simulink model "collision_avoidance_260310"  (R2024b)
settings: Solver=FixedStepAuto  StartTime=0.0  StopTime=inf  RelTol=1e-3  EnableMultiTasking=on
values from neighbouring files (symbols this model uses):
  Fx_max = 1    [Init_collision_avoidance_UGV.m]
  Fx_min = -1    [Init_collision_avoidance_UGV.m]
  N_max = 1    [Init_collision_avoidance_UGV.m]
  N_min = -1    [Init_collision_avoidance_UGV.m]
  RC_max = 2000    [Init_collision_avoidance_UGV.m]
  RC_min = 1000    [Init_collision_avoidance_UGV.m]
  ref_lla = [36.365227, 127.345838, 25.1110]    [Init_collision_avoidance_UGV.m]
undefined symbols (not defined in the file or in its folder): DiscIntNeverNeededParam, modeeight, modefive, modefour, modenine, modeone, modeseven, modesix, modeten, modethree, modetwo, motor_pwm_time_log, psi_time_log, r_time_log, rc_on_off, steering_pwm_time_log, taun_time_log, taux_time_log, timestamp, u_time_log, v_time_log, x_time_log, y_time_log
libraries: px4uORBlib x14, px4Utilslib x9, sharedtransform x2, sharedutil x1, px4Peripheralslib x1, px4Sensorslib x1
settings Model: ExtModeTrigDuration=10  Creator=ADMIN  LastModifiedBy=User
settings SolverCC: PositivePriorityOrder=on
settings OptimizationCC: EnhancedBackFolding=on  PassReuseOutputArgsAs=Individual arguments  ZeroExternalMemoryAtStartup=off  ZeroInternalMemoryAtStartup=off  MaxStackSize=64  OptimizeBlockOrder=speed  DifferentSizesBufferReuse=on  OptimizationCustomize=off  EfficientTunableParamExpr=on
settings DebuggingCC: ParameterTunabilityLossMsg=error
settings HardwareCC: ProdBitPerPointer=32  ProdBitPerSizeT=32  ProdBitPerPtrDiffT=32  ProdLargestAtomicInteger=Long  ProdLargestAtomicFloat=Double  ProdWordSize=32  ProdLongLongMode=on  ProdHWDeviceType=ARM Compatible->ARM Cortex
settings SFSimCC: MATLABDynamicMemAlloc=off  SimTargetLang=C++
settings RTWCC: Description=Embedded Coder  SystemTargetFile=ert.tlc  HardwareBoard=PX4 Pixhawk 6x  TLCOptions="-aInlineSetEventsForThisBaseRateFcn=TLC_FALSE -aSuppressMultiTaskScheduler=TLC_FALSE  -aRateBasedStepFcn=0"  TemplateMakefile=ert_default_tmf  Toolchain=GNU Tools for PX4 Autopilots  TargetLang=C++  GPUComputeCapability=3.5
settings CodeAppCC: ForceParamTrailComments=on  IgnoreCustomStorageClasses=off  OperatorAnnotations=on  SimulinkDataObjDesc=on  SFDataObjDesc=on  InsertBlockDesc=on
settings ERTTargetCC: ExtModeTransport=3  ExtModeStaticAlloc=on  ExtModeStaticAllocSize=1024  ExtModeMexFile=ext_xcp  ExtModeIntrfLevel=Level2 - Open  InlinedParameterPlacement=Hierarchical  DynamicArrayContainerType=coder::array

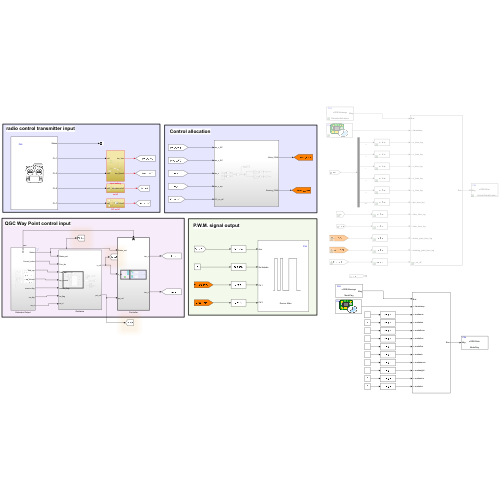
[thumbnail: Simulink's stored preview of the top-level diagram]
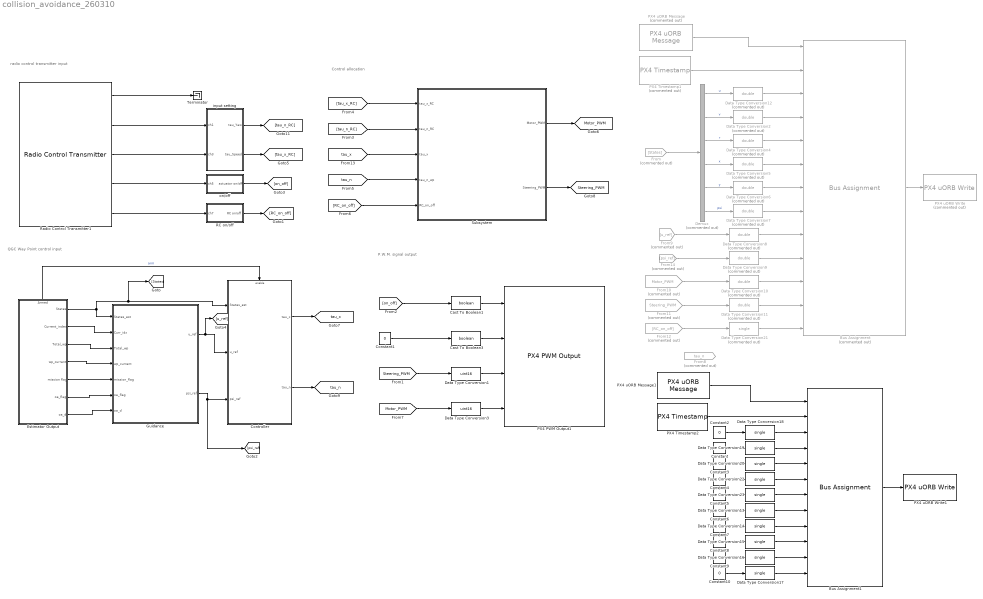
== system collision_avoidance_260310 ==
  note: radio control transmitter input
  note: P.W.M. signal output
  note: Control allocation
  note: QGC Way Point control input
  Bus Assignment : BusAssignment  Commented=on  AssignedSignals=timestamp,u_time_log,v_time_log,r_time_log,x_time_log,y_time_log,psi_time_log,taux_time_log,taun_time_log,motor_pwm_time_log,steering_pwm_time_log,rc_on_off
  Bus Assignment1 : BusAssignment  AssignedSignals=timestamp,modeone,modetwo,modethree,modefour,modefive,modesix,modeseven,modeeight,modenine,modeten
  Cast To Boolean1 : DataTypeConversion  OutDataTypeStr=boolean  SaturateOnIntegerOverflow=off  RndMeth=Floor
  Cast To Boolean3 : DataTypeConversion  OutDataTypeStr=boolean  SaturateOnIntegerOverflow=off  RndMeth=Floor
  Constant : Constant
  Constant{1..10} (10 alike) : Constant  Value=0
  Controller : Subsystem
  Data Type Conversion1 : DataTypeConversion  OutDataTypeStr=uint16  SaturateOnIntegerOverflow=off  RndMeth=Floor
  Data Type Conversion{2,4..12} (10 alike) : DataTypeConversion  Commented=on  OutDataTypeStr=double  RndMeth=Nearest  SaturateOnIntegerOverflow=off
  Data Type Conversion{13..20,22..23} (10 alike) : DataTypeConversion  OutDataTypeStr=single  RndMeth=Nearest  SaturateOnIntegerOverflow=off
  Data Type Conversion21 : DataTypeConversion  Commented=on  OutDataTypeStr=single  RndMeth=Nearest  SaturateOnIntegerOverflow=off
  Data Type Conversion3 : DataTypeConversion  OutDataTypeStr=uint16  SaturateOnIntegerOverflow=off  RndMeth=Floor
  Demux : Demux  Commented=on  Outputs=6
  Estimator Output : Subsystem
      settings: PortSchema="{\"entries\":[{\"content\":{\"sides\":[{\"content\":{},\"type\":\"ConnectorPlacement.EquallySpacedRectSide\",\"uuid\":\"1d36fcc8-80dd-4f77-9fb4-99d02af10106\"},{\"content\":{\"connectorIds\":[\"Out1\",\"Out2\",\"Out3\",\"Out4\",\"Out5\",\"Out6\",\"Out7\"],\"side\":\"RIGHT\"},\"type\":\"ConnectorPlacement.EquallySpacedRectSide\",\"uuid\":\"b131ae5f-f834-4065-827d-4788e597b476\"},{\"content\":{\"connectorIds\":[\"Out8\"],\"side\":\"TOP\"},\"type\":\"ConnectorPlacement.EquallySpacedRectSide\",\"uuid\":\"02aebafc-cadb-49e7-bb89-79250ef56f49\"}]},\"type\":\"ConnectorPlacement.EquallySpacedConnector\",\"uuid\":\"ac2ee399-74d4-4a66-adbe-2c3e3c8a8081\"}],\"packageUris\":[\"http://schema.mathworks.com/mf0/Connector/R2020b\"],\"version\":\"1.0\"}"
  From : From  Commented=on  GotoTag=States
  From10 : From  Commented=on  GotoTag=Motor_PWM  TagVisibility=global
  From11 : From  Commented=on  GotoTag=Steering_PWM  TagVisibility=global
  From12 : From  Commented=on  GotoTag=RC_on_off
  From14 : From  Commented=on  GotoTag=psi_ref
  From8 : From  Commented=on  GotoTag=tau_n  TagVisibility=global
  From9 : From  Commented=on  GotoTag=u_ref
  "Guidance " : Subsystem
  PX4 PWM Output1 : px4Peripheralslib/PX4 PWM Output  pwmDevice=Main  pwmChannel1_=on  pwmChannel2_=off  pwmChannel3_=on  pwmChannel4_=off  pwmChannel5_=off  pwmChannel6_=off  pwmChannel7_=off  pwmChannel8_=off
      settings: SourceProductName=PX4 Peripheral Blocks
  PX4 Timestamp1 : px4Utilslib/PX4 Timestamp  Commented=on  SampleTime=-1
      settings: SourceProductName=PX4 Utility Blocks
  PX4 Timestamp2 : px4Utilslib/PX4 Timestamp  SampleTime=-1
      settings: SourceProductName=PX4 Utility Blocks
  PX4 uORB Message : px4uORBlib/PX4 uORB Message  Commented=on  uORBTopic=StatesAndActuators  SampleTime=-1  selectInstance=StatesAndActuators
  PX4 uORB Message1 : px4uORBlib/PX4 uORB Message  uORBTopic=ModeFlag  SampleTime=-1  selectInstance=ModeFlag
  PX4 uORB Write : px4uORBlib/PX4 uORB Write  Commented=on  uORBTopic=VehicleGlobalPosition  selectInstance=vehicle_global_position  MessageQueueLen=1
  PX4 uORB Write1 : px4uORBlib/PX4 uORB Write  uORBTopic=ModeFlag  selectInstance=ModeFlag  MessageQueueLen=1
  RC on/off : Subsystem
  Radio Control Transmitter1 : px4Sensorslib/Radio Control Transmitter  channel1=on  channel2=off  channel3=on  channel4=off  channel5=on  channel6=off  channel7=on  channel8=off  channel_count=off  rssi=off  rc_input_source=off  timestamp_last_signal=off  time_stamp=off  sampleTime=1/250  BlockingMode=off  BlockTimeout=5
  Subsystem : Subsystem
  Terminator : Terminator
  input setting : Subsystem
  on/off : Subsystem
  tag scope: Motor_PWM=global, Steering_PWM=global, tau_n=global, tau_x=global
  wires:
  [tau_n_RC] -> Subsystem/2(tau_n_RC)
  Radio Control Transmitter1/3 -> input setting/2(ch3)
  on/off/1(actuator on/off) -> [on_off]
  Radio Control Transmitter1/1 -> Terminator/1
  Radio Control Transmitter1/4 -> on/off/1(ch5)
  [on_off] -> Cast To Boolean1/1
  Constant1/1 -> Cast To Boolean3/1
  Radio Control Transmitter1/5 -> RC on/off/1(ch7)
  RC on/off/1(RC on/off) -> [RC_on_off]
  input setting/1(tau_Yaw) -> [tau_n_RC]
  input setting/2(tau_Speed) -> [tau_x_RC]
  Radio Control Transmitter1/2 -> input setting/1(ch1)
  [tau_x] -> Subsystem/3(tau_x)
  [RC_on_off] -> Subsystem/5(RC_on_off)
  [tau_n] -> Subsystem/4(tau_n_wp)
  Cast To Boolean1/1 -> PX4 PWM Output1/1
  Cast To Boolean3/1 -> PX4 PWM Output1/2
  Data Type Conversion1/1 -> PX4 PWM Output1/3
  Data Type Conversion3/1 -> PX4 PWM Output1/4
  Subsystem/1(Motor_PWM) -> [Motor_PWM]
  Subsystem/2(Steering_PWM) -> [Steering_PWM]
  [Steering_PWM] -> Data Type Conversion1/1
  [Motor_PWM] -> Data Type Conversion3/1
  Estimator Output/4(wp_current) -> "Guidance "/4(wp_current)
  Estimator Output/3(Total_wp) -> "Guidance "/3(Total_wp)
  Estimator Output/2(Current_index) -> "Guidance "/2(Curr_idx)
  Estimator Output/1(States) -> [States], Controller/1(States_est), "Guidance "/1(States_est)
  Estimator Output/5(mission flag) -> "Guidance "/5(mission_flag)
  "Guidance "/1(u_ref) -> Controller/2(u_ref), [u_ref]
  "Guidance "/2(psi_ref) -> [psi_ref], Controller/3(psi_ref)
  Controller/2(tau_n) -> [tau_n]
  Controller/1(tau_x) -> [tau_x]
  [tau_x_RC] -> Subsystem/1(tau_x_RC)
  Estimator Output/8(Armed) -> Controller/Enable  "arm"
  From/1 -> Demux/1
  Demux/1 -> Data Type Conversion12/1  "u"
  Demux/2 -> Data Type Conversion2/1  "v"
  Demux/3 -> Data Type Conversion4/1  "r"
  Demux/4 -> Data Type Conversion5/1  "x"
  Demux/5 -> Data Type Conversion6/1  "y"
  Demux/6 -> Data Type Conversion7/1  "psi"
  From9/1 -> Data Type Conversion8/1
  From14/1 -> Data Type Conversion9/1
  From10/1 -> Data Type Conversion10/1
  From11/1 -> Data Type Conversion11/1
  Constant6/1 -> Data Type Conversion13/1
  Data Type Conversion23/1 -> Bus Assignment1/7
  Constant8/1 -> Data Type Conversion15/1
  Constant9/1 -> Data Type Conversion16/1
  Data Type Conversion19/1 -> Bus Assignment1/4
  Data Type Conversion15/1 -> Bus Assignment1/10
  Constant/1 -> Data Type Conversion19/1
  Data Type Conversion16/1 -> Bus Assignment1/11
  Constant2/1 -> Data Type Conversion18/1
  Constant3/1 -> Data Type Conversion20/1
  Data Type Conversion17/1 -> Bus Assignment1/12
  Data Type Conversion18/1 -> Bus Assignment1/3
  Data Type Conversion13/1 -> Bus Assignment1/8
  Data Type Conversion14/1 -> Bus Assignment1/9
  Data Type Conversion22/1 -> Bus Assignment1/6
  Constant5/1 -> Data Type Conversion23/1
  Constant4/1 -> Data Type Conversion22/1
  Constant7/1 -> Data Type Conversion14/1
  Constant10/1 -> Data Type Conversion17/1
  Data Type Conversion20/1 -> Bus Assignment1/5
  PX4 uORB Message/1 -> Bus Assignment/1
  PX4 Timestamp1/1 -> Bus Assignment/2
  From12/1 -> Data Type Conversion21/1
  Data Type Conversion11/1 -> Bus Assignment/12
  Data Type Conversion10/1 -> Bus Assignment/11
  Data Type Conversion9/1 -> Bus Assignment/10
  Data Type Conversion8/1 -> Bus Assignment/9
  Data Type Conversion7/1 -> Bus Assignment/8
  Data Type Conversion6/1 -> Bus Assignment/7
  Data Type Conversion5/1 -> Bus Assignment/6
  Data Type Conversion4/1 -> Bus Assignment/5
  Data Type Conversion2/1 -> Bus Assignment/4
  Data Type Conversion12/1 -> Bus Assignment/3
  Bus Assignment/1 -> PX4 uORB Write/1
  PX4 uORB Message1/1 -> Bus Assignment1/1
  PX4 Timestamp2/1 -> Bus Assignment1/2
  Bus Assignment1/1 -> PX4 uORB Write1/1
  Estimator Output/6(oa_flag) -> "Guidance "/6(oa_flag)
  Estimator Output/7(oa_d) -> "Guidance "/7(oa_d)
  Data Type Conversion21/1 -> Bus Assignment/13

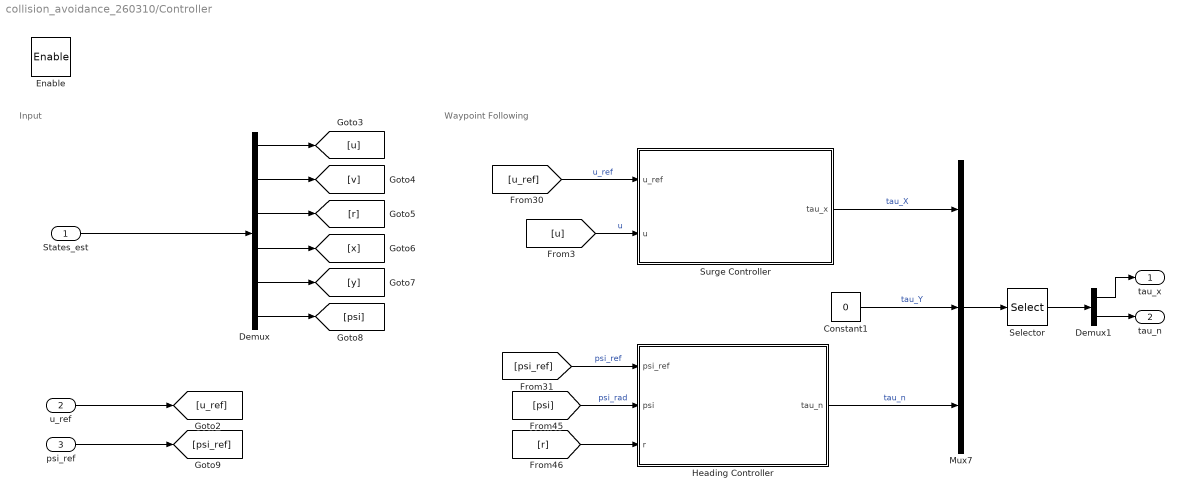
== system collision_avoidance_260310/Controller ==
  note: Input
  note: Waypoint Following
  States_est : Inport
  u_ref : Inport  Port=2
  psi_ref : Inport  Port=3
  Enable : EnablePort
  Constant1 : Constant  Value=0
  Demux : Demux  Outputs=6
  Demux1 : Demux  Outputs=2
  Heading Controller : Subsystem
  Mux7 : Mux  Inputs=3
  Selector : Selector  InputPortWidth=3  IndexOptions=Index vector (dialog)  Indices=[1 3]  OutputSizes=1
  Surge Controller : Subsystem
  tau_x : Outport
  tau_n : Outport  Port=2
  wires:
  Surge Controller/1(tau_x) -> Mux7/1  "tau_X"
  Constant1/1 -> Mux7/2  "tau_Y"
  [psi_ref] -> Heading Controller/1(psi_ref)  "psi_ref"
  [r] -> Heading Controller/3(r)
  Mux7/1 -> Selector/1
  States_est/1 -> Demux/1
  Demux/1 -> [u]
  Demux/2 -> [v]
  Demux/3 -> [r]
  Demux/4 -> [x]
  Demux/5 -> [y]
  Demux/6 -> [psi]
  u_ref/1 -> [u_ref]
  psi_ref/1 -> [psi_ref]
  [u_ref] -> Surge Controller/1(u_ref)  "u_ref"
  [u] -> Surge Controller/2(u)  "u"
  Heading Controller/1(tau_n) -> Mux7/3  "tau_n"
  [psi] -> Heading Controller/2(psi)  "psi_rad"
  Selector/1 -> Demux1/1
  Demux1/1 -> tau_x/1
  Demux1/2 -> tau_n/1

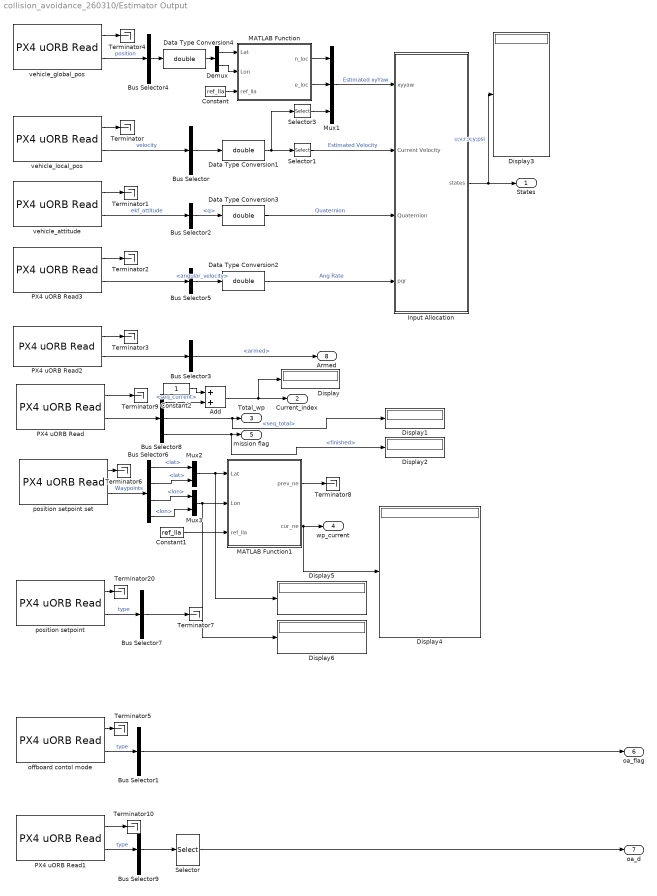
== system collision_avoidance_260310/Estimator Output ==
  Add : Sum
  Bus Selector : BusSelector  OutputSignals=vx,vy,vz,heading  OutputAsBus=on
  Bus Selector1 : BusSelector  OutputSignals=position,velocity,attitude  OutputAsBus=on
  Bus Selector2 : BusSelector  OutputSignals=q
  Bus Selector3 : BusSelector  OutputSignals=armed
  Bus Selector4 : BusSelector  OutputSignals=lat,lon  OutputAsBus=on
  Bus Selector5 : BusSelector  OutputSignals=angular_velocity
  Bus Selector6 : BusSelector  OutputSignals=previous.lat,current.lat,previous.lon,current.lon
  Bus Selector7 : BusSelector  OutputSignals=type  OutputAsBus=on
  Bus Selector8 : BusSelector  OutputSignals=seq_current,seq_total,finished
  Bus Selector9 : BusSelector  OutputSignals=position,velocity,yaw  OutputAsBus=on
  Constant : Constant  Value=ref_lla  VectorParams1D=off
  Constant1 : Constant  Value=ref_lla  VectorParams1D=off
  Constant2 : Constant
  Data Type Conversion{1..4} (4 alike) : DataTypeConversion  OutDataTypeStr=double  SaturateOnIntegerOverflow=off  RndMeth=Floor
  Demux : Demux  Outputs=2
  Display{,1..6} (7 alike) : Display
  Input Allocation : Subsystem
  MATLAB Function : MATLAB Function  TreatAsAtomicUnit=on
  MATLAB Function1 : MATLAB Function  TreatAsAtomicUnit=on
  Mux1 : Mux  Inputs=3
  Mux2 : Mux  Inputs=2
  Mux3 : Mux  Inputs=2
  PX4 uORB Read : px4uORBlib/PX4 uORB Read  uORBTopic=MissionResult  selectInstance=MissionResult  SampleTime=-1  BlockingMode=off  BlockTimeout=1e-3
  PX4 uORB Read1 : px4uORBlib/PX4 uORB Read  uORBTopic=TrajectorySetpoint  selectInstance=TrajectorySetpoint  SampleTime=-1  BlockingMode=off  BlockTimeout=1e-3
  PX4 uORB Read2 : px4uORBlib/PX4 uORB Read  uORBTopic=ActuatorArmed  selectInstance=ActuatorArmed  SampleTime=-1  BlockingMode=off  BlockTimeout=1e-3
  PX4 uORB Read3 : px4uORBlib/PX4 uORB Read  uORBTopic=VehicleOdometry  selectInstance=vehicle_odometry  SampleTime=-1  BlockingMode=off  BlockTimeout=1e-3
  Selector : Selector  InputPortWidth=7  IndexOptions=Index vector (dialog)  Indices=[1:7]  OutputSizes=1
  Selector1 : Selector  InputPortWidth=4  IndexOptions=Index vector (dialog)  Indices=[1:3]  OutputSizes=1
  Selector3 : Selector  InputPortWidth=4  IndexOptions=Index vector (dialog)  Indices=4  OutputSizes=1
  Terminator{,1..10,20} (12 alike) : Terminator
  offboard contol mode : px4uORBlib/PX4 uORB Read  uORBTopic=OffboardControlMode  selectInstance=OffboardControlMode  SampleTime=-1  BlockingMode=off  BlockTimeout=1e-3
  position setpoint : px4uORBlib/PX4 uORB Read  uORBTopic=PositionSetpoint  selectInstance=PositionSetpoint  SampleTime=-1  BlockingMode=off  BlockTimeout=1e-3
  position setpoint set : px4uORBlib/PX4 uORB Read  uORBTopic=PositionSetpointTriplet  selectInstance=PositionSetpointTriplet  SampleTime=-1  BlockingMode=off  BlockTimeout=1e-3
  vehicle_attitude : px4uORBlib/PX4 uORB Read  uORBTopic=VehicleAttitude  selectInstance=vehicle_attitude  SampleTime=-1  BlockingMode=off  BlockTimeout=1e-3
  vehicle_global_pos : px4uORBlib/PX4 uORB Read  uORBTopic=VehicleGlobalPosition  selectInstance=vehicle_global_position  SampleTime=-1  BlockingMode=off  BlockTimeout=1e-3
  vehicle_local_pos : px4uORBlib/PX4 uORB Read  uORBTopic=VehicleLocalPosition  selectInstance=vehicle_local_position  SampleTime=-1  BlockingMode=off  BlockTimeout=1e-3
  States : Outport
  Current_index : Outport  Port=2
  Total_wp : Outport  Port=3
  wp_current : Outport  Port=4
  mission flag : Outport  Port=5
  oa_flag : Outport  Port=6
  oa_d : Outport  Port=7
  Armed : Outport  Port=8
  wires:
  PX4 uORB Read3/1 -> Terminator2/1
  Data Type Conversion2/1 -> Input Allocation/4(pqr)  "Ang Rate"
  Data Type Conversion3/1 -> Input Allocation/3(Quaternion)  "Quaternion"
  Bus Selector2/1 -> Data Type Conversion3/1  "<q>"
  Mux1/1 -> Input Allocation/1(xyyaw)  "Estimated xyYaw"
  Selector3/1 -> Mux1/3
  vehicle_local_pos/1 -> Terminator/1
  vehicle_global_pos/2 -> Bus Selector4/1  "position"
  Bus Selector/1 -> Data Type Conversion1/1
  MATLAB Function/1(n_loc) -> Mux1/1
  vehicle_attitude/1 -> Terminator1/1
  Selector1/1 -> Input Allocation/2(Current Velocity)  "Estimated Velocity"
  vehicle_attitude/2 -> Bus Selector2/1  "ekf_attitude"
  vehicle_local_pos/2 -> Bus Selector/1  "velocity"
  Bus Selector4/1 -> Data Type Conversion4/1
  MATLAB Function/2(e_loc) -> Mux1/2
  Data Type Conversion1/1 -> Selector3/1, Selector1/1
  vehicle_global_pos/1 -> Terminator4/1
  PX4 uORB Read2/2 -> Bus Selector3/1
  Bus Selector3/1 -> Armed/1  "<armed>"
  PX4 uORB Read2/1 -> Terminator3/1
  Demux/1 -> MATLAB Function/1(Lat)
  Constant/1 -> MATLAB Function/3(ref_lla)
  Data Type Conversion4/1 -> Demux/1
  Demux/2 -> MATLAB Function/2(Lon)
  Input Allocation/1(states) -> Display3/1, States/1  "u;v;r;x;y;psi"
  Bus Selector7/1 -> Terminator7/1
  position setpoint/2 -> Bus Selector7/1  "type"
  position setpoint set/2 -> Bus Selector6/1  "Waypoints"
  Mux3/1 -> Display6/1, MATLAB Function1/2(Lon)
  Bus Selector6/4 -> Mux3/2  "<lon>"
  MATLAB Function1/1(prev_ne) -> Terminator8/1
  Bus Selector6/3 -> Mux3/1  "<lon>"
  Bus Selector6/1 -> Mux2/1  "<lat>"
  Mux2/1 -> Display5/1, MATLAB Function1/1(Lat)
  position setpoint/1 -> Terminator20/1
  Bus Selector6/2 -> Mux2/2  "<lat>"
  MATLAB Function1/2(cur_ne) -> Display4/1, wp_current/1
  position setpoint set/1 -> Terminator6/1
  Constant1/1 -> MATLAB Function1/3(ref_lla)
  PX4 uORB Read/2 -> Bus Selector8/1
  PX4 uORB Read/1 -> Terminator9/1
  Bus Selector8/2 -> Display1/1, Total_wp/1  "<seq_total>"
  Bus Selector8/3 -> Display2/1, mission flag/1  "<finished>"
  Bus Selector8/1 -> Add/2  "<seq_current>"
  Constant2/1 -> Add/1
  Add/1 -> Display/1, Current_index/1
  PX4 uORB Read3/2 -> Bus Selector5/1
  Bus Selector5/1 -> Data Type Conversion2/1  "<angular_velocity>"
  offboard contol mode/1 -> Terminator5/1
  PX4 uORB Read1/2 -> Bus Selector9/1  "type"
  Bus Selector9/1 -> Selector/1
  Bus Selector1/1 -> oa_flag/1
  offboard contol mode/2 -> Bus Selector1/1  "type"
  PX4 uORB Read1/1 -> Terminator10/1
  Selector/1 -> oa_d/1

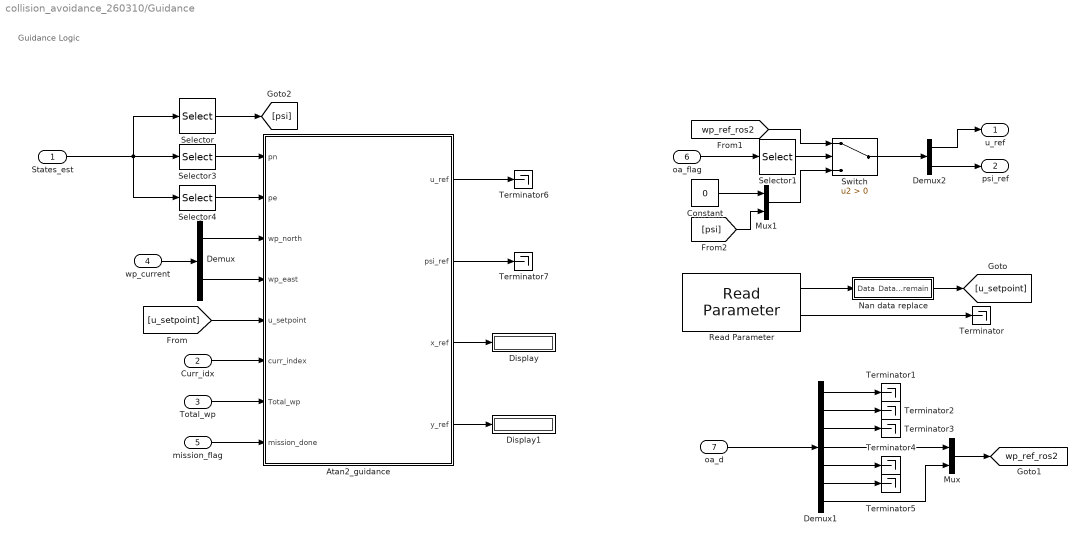
== system collision_avoidance_260310/Guidance  ==
  note: Guidance Logic
  States_est : Inport
  Curr_idx : Inport  Port=2
  Total_wp : Inport  Port=3
  wp_current : Inport  Port=4
  mission_flag : Inport  Port=5
  oa_flag : Inport  Port=6
  oa_d : Inport  Port=7
  Atan2_guidance : MATLAB Function  TreatAsAtomicUnit=on
  Constant : Constant  Value=0
  Demux : Demux  Outputs=2
  Demux1 : Demux  Outputs=7
  Demux2 : Demux  Outputs=2
  Display : Display
  Display1 : Display
  Mux : Mux  Inputs=2
  Mux1 : Mux  Inputs=2
  Nan data replace : Subsystem
  Read Parameter : px4Utilslib/Read Parameter  ParameterName=SURGE_VEL_SETP  DataType=FLOAT  SampleTime=-1
      settings: SourceProductName=PX4 Utility Blocks
  Selector : Selector  InputPortWidth=6  IndexOptions=Index vector (dialog)  Indices=6  OutputSizes=1
  Selector1 : Selector  InputPortWidth=3  IndexOptions=Index vector (dialog)  Indices=2  OutputSizes=1
  Selector3 : Selector  InputPortWidth=6  IndexOptions=Index vector (dialog)  Indices=4  OutputSizes=1
  Selector4 : Selector  InputPortWidth=6  IndexOptions=Index vector (dialog)  Indices=5  OutputSizes=1
  Switch : Switch  Criteria=u2 > Threshold  SaturateOnIntegerOverflow=off  InputSameDT=off
  Terminator{,1..7} (8 alike) : Terminator
  u_ref : Outport
  psi_ref : Outport  Port=2
  tag scope: wp_ref_ros2=global
  wires:
  Total_wp/1 -> Atan2_guidance/7(Total_wp)
  Selector4/1 -> Atan2_guidance/2(pe)
  States_est/1 -> Selector/1, Selector4/1, Selector3/1
  Selector3/1 -> Atan2_guidance/1(pn)
  Demux/1 -> Atan2_guidance/3(wp_north)
  Demux/2 -> Atan2_guidance/4(wp_east)
  Atan2_guidance/3(x_ref) -> Display/1
  Atan2_guidance/4(y_ref) -> Display1/1
  Curr_idx/1 -> Atan2_guidance/6(curr_index)
  mission_flag/1 -> Atan2_guidance/8(mission_done)
  wp_current/1 -> Demux/1
  Read Parameter/2 -> Terminator/1
  [u_setpoint] -> Atan2_guidance/5(u_setpoint)
  Read Parameter/1 -> Nan data replace/1(Data)
  Nan data replace/1(Data_remain) -> [u_setpoint]
  oa_flag/1 -> Selector1/1
  oa_d/1 -> Demux1/1
  Demux1/1 -> Terminator1/1
  Demux1/2 -> Terminator2/1
  Demux1/3 -> Terminator3/1
  Demux1/5 -> Terminator4/1
  Demux1/6 -> Terminator5/1
  Demux1/4 -> Mux/1
  Demux1/7 -> Mux/2
  Switch/1 -> Demux2/1
  Demux2/2 -> psi_ref/1
  Demux2/1 -> u_ref/1
  Mux/1 -> [wp_ref_ros2]
  [wp_ref_ros2] -> Switch/1
  Mux1/1 -> Switch/3
  Atan2_guidance/1(u_ref) -> Terminator6/1
  Atan2_guidance/2(psi_ref) -> Terminator7/1
  Selector/1 -> [psi]
  [psi] -> Mux1/2
  Constant/1 -> Mux1/1
  Selector1/1 -> Switch/2

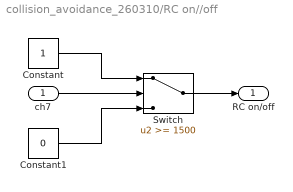
== system collision_avoidance_260310/RC on//off ==
  ch7 : Inport
  Constant : Constant
  Constant1 : Constant  Value=0
  Switch : Switch  Threshold=1500  SaturateOnIntegerOverflow=off  InputSameDT=off
  RC on/off : Outport
  wires:
  Switch/1 -> RC on/off/1
  ch7/1 -> Switch/2
  Constant/1 -> Switch/1
  Constant1/1 -> Switch/3

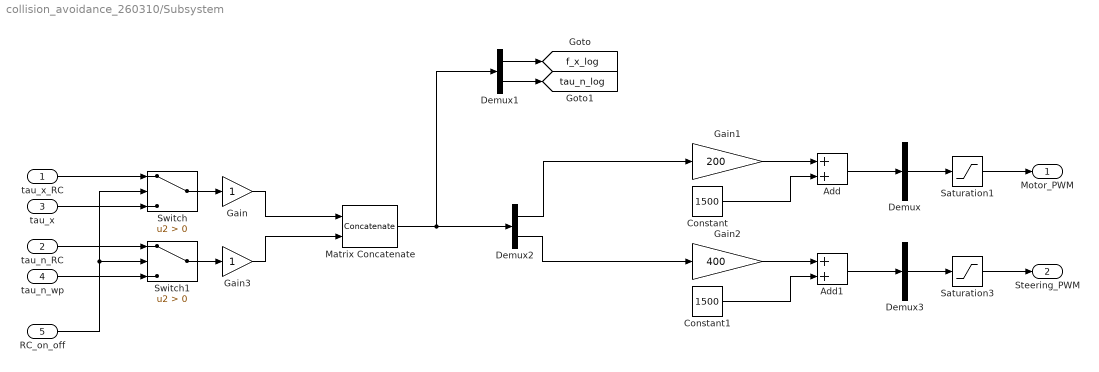
== system collision_avoidance_260310/Subsystem ==
  tau_x_RC : Inport
  tau_n_RC : Inport  Port=2
  tau_x : Inport  Port=3
  tau_n_wp : Inport  Port=4
  RC_on_off : Inport  Port=5
  Add : Sum
  Add1 : Sum
  Constant : Constant  Value=1500
  Constant1 : Constant  Value=1500
  Demux : Demux  Outputs=1
  Demux1 : Demux  Outputs=2
  Demux2 : Demux  Outputs=2
  Demux3 : Demux  Outputs=1
  Gain : Gain
  Gain1 : Gain  Gain=200
  Gain2 : Gain  Gain=400
  Gain3 : Gain
  Matrix Concatenate : Concatenate  Mode=Multidimensional array
  Saturation1 : Saturate  UpperLimit=2000  LowerLimit=1000
  Saturation3 : Saturate  UpperLimit=2000  LowerLimit=1000
  Switch : Switch  Criteria=u2 > Threshold  SaturateOnIntegerOverflow=off  InputSameDT=off
  Switch1 : Switch  Criteria=u2 > Threshold  SaturateOnIntegerOverflow=off  InputSameDT=off
  Motor_PWM : Outport
  Steering_PWM : Outport  Port=2
  tag scope: f_x_log=global, tau_n_log=global
  wires:
  RC_on_off/1 -> Switch1/2, Switch/2
  tau_x_RC/1 -> Switch/1
  tau_x/1 -> Switch/3
  tau_n_RC/1 -> Switch1/1
  tau_n_wp/1 -> Switch1/3
  Switch/1 -> Gain/1
  Switch1/1 -> Gain3/1
  Demux1/1 -> [f_x_log]
  Demux1/2 -> [tau_n_log]
  Demux3/1 -> Saturation3/1
  Gain1/1 -> Add/1
  Matrix Concatenate/1 -> Demux2/1, Demux1/1
  Demux2/1 -> Gain1/1
  Constant/1 -> Add/2
  Add1/1 -> Demux3/1
  Saturation3/1 -> Steering_PWM/1
  Demux2/2 -> Gain2/1
  Constant1/1 -> Add1/2
  Add/1 -> Demux/1
  Demux/1 -> Saturation1/1
  Gain2/1 -> Add1/1
  Saturation1/1 -> Motor_PWM/1
  Gain/1 -> Matrix Concatenate/1
  Gain3/1 -> Matrix Concatenate/2

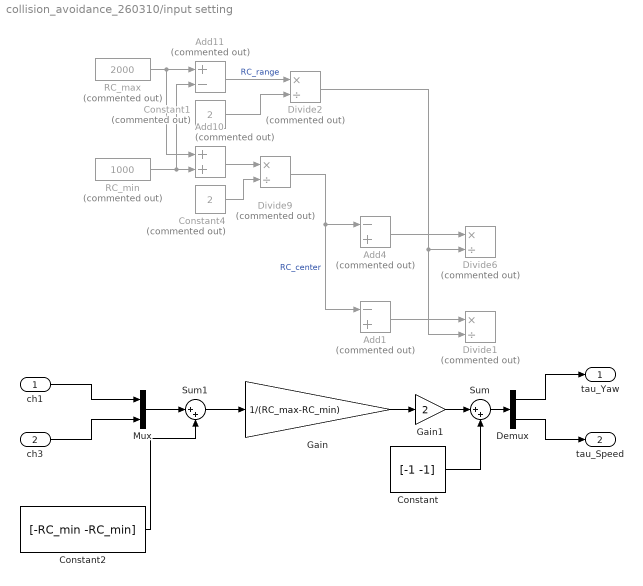
== system collision_avoidance_260310/input setting ==
  ch1 : Inport
  ch3 : Inport  Port=2
  Add1 : Sum  Commented=on  Inputs=-+  OutDataTypeStr=single
  Add10 : Sum  Commented=on
  Add11 : Sum  Commented=on  Inputs=+-
  Add4 : Sum  Commented=on  Inputs=-+  OutDataTypeStr=single
  Constant : Constant  Value=[-1 -1]
  Constant1 : Constant  Commented=on  Value=2  OutDataTypeStr=single
  Constant2 : Constant  Value=[-RC_min -RC_min]
  Constant4 : Constant  Commented=on  Value=2  OutDataTypeStr=single
  Demux : Demux  Outputs=2
  Divide{1..2,6,9} (4 alike) : Product  Commented=on  Inputs=*/
  Gain : Gain  Gain=1/(RC_max-RC_min)
  Gain1 : Gain  Gain=2
  Mux : Mux  Inputs=2
  RC_max : Constant  Commented=on  Value=2000  OutDataTypeStr=int16
  RC_min : Constant  Commented=on  Value=1000  OutDataTypeStr=int16
  Sum : Sum  Inputs=|++
  Sum1 : Sum  Inputs=|++
  tau_Yaw : Outport
  tau_Speed : Outport  Port=2
  wires:
  Constant4/1 -> Divide9/2
  Add10/1 -> Divide9/1
  Constant1/1 -> Divide2/2
  Add11/1 -> Divide2/1  "RC_range"
  RC_max/1 -> Add10/1, Add11/1
  RC_min/1 -> Add11/2, Add10/2
  ch1/1 -> Mux/1
  Divide9/1 -> Add1/1, Add4/1  "RC_center"
  Add4/1 -> Divide6/1
  Divide2/1 -> Divide1/2, Divide6/2
  ch3/1 -> Mux/2
  Add1/1 -> Divide1/1
  Gain/1 -> Gain1/1
  Mux/1 -> Sum1/1
  Gain1/1 -> Sum/1
  Sum1/1 -> Gain/1
  Sum/1 -> Demux/1
  Demux/1 -> tau_Yaw/1
  Demux/2 -> tau_Speed/1
  Constant/1 -> Sum/2
  Constant2/1 -> Sum1/2

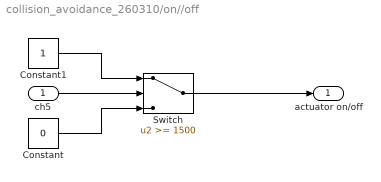
== system collision_avoidance_260310/on//off ==
  ch5 : Inport
  Constant : Constant  Value=0
  Constant1 : Constant
  Switch : Switch  Threshold=1500  SaturateOnIntegerOverflow=off  InputSameDT=off
  actuator on/off : Outport
  wires:
  Constant1/1 -> Switch/1
  Constant/1 -> Switch/3
  ch5/1 -> Switch/2
  Switch/1 -> actuator on/off/1

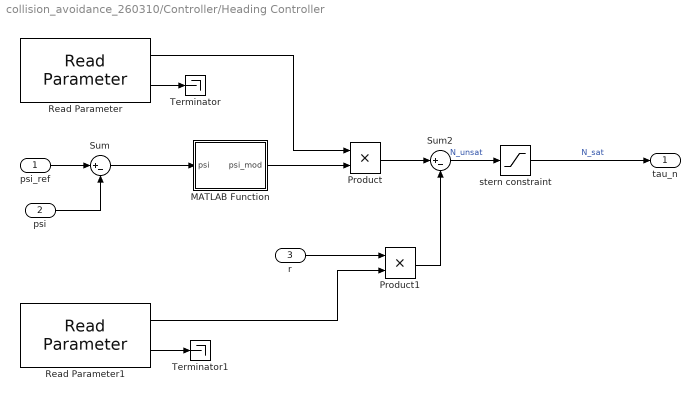
== system collision_avoidance_260310/Controller/Heading Controller ==
  psi_ref : Inport
  psi : Inport  Port=2
  r : Inport  Port=3
  MATLAB Function : MATLAB Function  TreatAsAtomicUnit=on
  Product : Product
  Product1 : Product
  Read Parameter : px4Utilslib/Read Parameter  ParameterName=HEADING_P  DataType=FLOAT  SampleTime=-1
      settings: SourceProductName=PX4 Utility Blocks
  Read Parameter1 : px4Utilslib/Read Parameter  ParameterName=HEADING_D  DataType=FLOAT  SampleTime=-1
      settings: SourceProductName=PX4 Utility Blocks
  Sum : Sum  Inputs=|+-
  Sum2 : Sum  Inputs=|+-  InputSameDT=on  SaturateOnIntegerOverflow=on  OutDataTypeStr=Inherit: Same as first input
  Terminator : Terminator
  Terminator1 : Terminator
  stern constraint : Saturate  UpperLimit=N_max  LowerLimit=N_min
      settings: AttributesFormatString=%<LowerLimit>~%<UpperLimit>
  tau_n : Outport
  wires:
  Sum/1 -> MATLAB Function/1(psi)
  Product/1 -> Sum2/1
  Sum2/1 -> stern constraint/1  "N_unsat"
  Product1/1 -> Sum2/2
  r/1 -> Product1/1
  stern constraint/1 -> tau_n/1  "N_sat"
  psi_ref/1 -> Sum/1
  psi/1 -> Sum/2
  MATLAB Function/1(psi_mod) -> Product/2
  Read Parameter/2 -> Terminator/1
  Read Parameter/1 -> Product/1
  Read Parameter1/1 -> Product1/2
  Read Parameter1/2 -> Terminator1/1

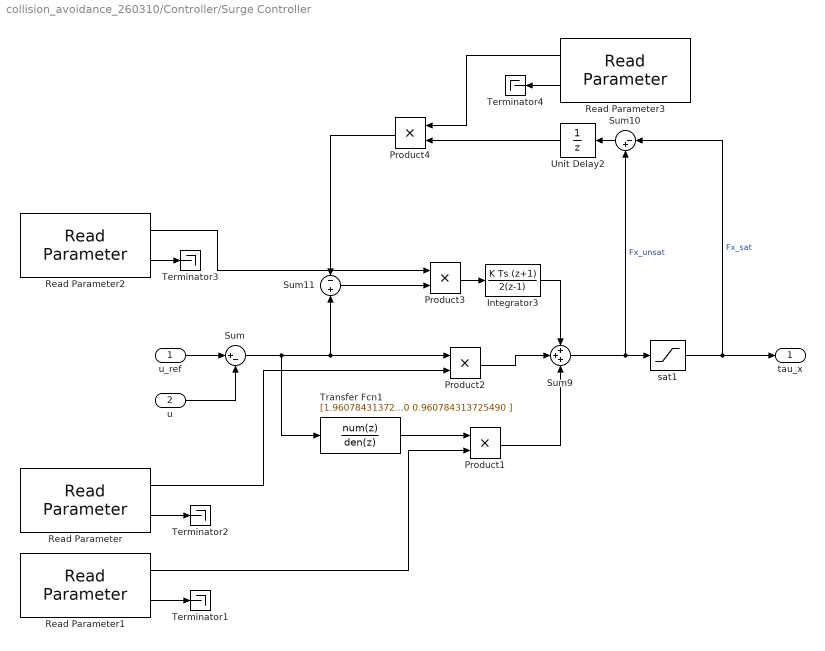
== system collision_avoidance_260310/Controller/Surge Controller ==
  u_ref : Inport
  u : Inport  Port=2
  Integrator3 : DiscreteIntegrator  IntegratorMethod=Integration: Trapezoidal  SampleTime=-1  ICPrevOutput=DiscIntNeverNeededParam  ICPrevScaledInput=DiscIntNeverNeededParam  mask(DiscretizedDiscreteIntegrator){}
      mask init:
      | %tustin
  Product{1..4} (4 alike) : Product
  Read Parameter : px4Utilslib/Read Parameter  ParameterName=SURGE_VEL_P  DataType=FLOAT  SampleTime=-1
      settings: SourceProductName=PX4 Utility Blocks
  Read Parameter1 : px4Utilslib/Read Parameter  ParameterName=SURGE_VEL_D  DataType=FLOAT  SampleTime=-1
      settings: SourceProductName=PX4 Utility Blocks
  Read Parameter2 : px4Utilslib/Read Parameter  ParameterName=SURGE_VEL_I  DataType=FLOAT  SampleTime=-1
      settings: SourceProductName=PX4 Utility Blocks
  Read Parameter3 : px4Utilslib/Read Parameter  ParameterName=SURGE_VEL_KANTI  DataType=FLOAT  SampleTime=-1
      settings: SourceProductName=PX4 Utility Blocks
  Sum : Sum  Inputs=|+-
  Sum10 : Sum  Inputs=|-+  InputSameDT=on  SaturateOnIntegerOverflow=on  OutDataTypeStr=Inherit: Same as first input
  Sum11 : Sum  Inputs=-|+  InputSameDT=on  SaturateOnIntegerOverflow=on  OutDataTypeStr=Inherit: Same as first input
  Sum9 : Sum  Inputs=+++  InputSameDT=on  SaturateOnIntegerOverflow=on  OutDataTypeStr=Inherit: Same as first input
  Terminator{1..4} (4 alike) : Terminator
  Transfer Fcn1 : DiscreteTransferFcn  Numerator=[1.960784313725490 -1.960784313725490 ]  Denominator=[1.000000000000000 0.960784313725490 ]  mask(DiscretizedDiscreteTransferFcn){}
      mask init:
      | %tustin
  Unit Delay2 : UnitDelay  SampleTime=-1  HasFrameUpgradeWarning=on
  sat1 : Saturate  UpperLimit=Fx_max  LowerLimit=Fx_min
      settings: AttributesFormatString=%<LowerLimit>~%<UpperLimit>
  tau_x : Outport
  wires:
  Sum11/1 -> Product3/2
  sat1/1 -> tau_x/1, Sum10/1  "Fx_sat"
  Product1/1 -> Sum9/3
  Integrator3/1 -> Sum9/1
  Sum/1 -> Product2/1, Sum11/2, Transfer Fcn1/1
  Transfer Fcn1/1 -> Product1/1
  Sum10/1 -> Unit Delay2/1
  Sum9/1 -> sat1/1, Sum10/2  "Fx_unsat"
  Product3/1 -> Integrator3/1
  Product4/1 -> Sum11/1
  Product2/1 -> Sum9/2
  u_ref/1 -> Sum/1
  u/1 -> Sum/2
  Unit Delay2/1 -> Product4/2
  Read Parameter1/2 -> Terminator1/1
  Read Parameter1/1 -> Product1/2
  Read Parameter/2 -> Terminator2/1
  Read Parameter/1 -> Product2/2
  Read Parameter2/2 -> Terminator3/1
  Read Parameter2/1 -> Product3/1
  Read Parameter3/2 -> Terminator4/1
  Read Parameter3/1 -> Product4/1

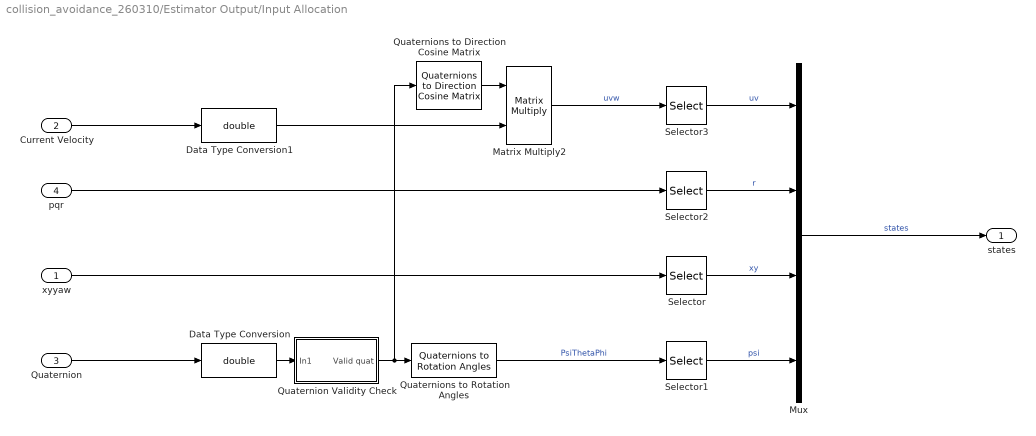
== system collision_avoidance_260310/Estimator Output/Input Allocation ==
  xyyaw : Inport
  Current Velocity : Inport  Port=2
  Quaternion : Inport  Port=3
  pqr : Inport  Port=4
  Data Type Conversion : DataTypeConversion  OutDataTypeStr=double  SaturateOnIntegerOverflow=off  RndMeth=Floor
  Data Type Conversion1 : DataTypeConversion  OutDataTypeStr=double  SaturateOnIntegerOverflow=off  RndMeth=Floor
  Matrix Multiply2 : Product  Multiplication=Matrix(*)
  Mux : Mux
  Quaternion Validity Check : Subsystem
  Quaternions to Direction Cosine Matrix : sharedtransform/Quaternions to  Direction Cosine Matrix  aMode=aMode
  Quaternions to Rotation Angles : sharedtransform/Quaternions to Rotation Angles  rotationOrder=ZYX  aMode=aMode
  Selector : Selector  InputPortWidth=3  IndexOptions=Index vector (dialog)  Indices=[1:2]  OutputSizes=1
  Selector1 : Selector  InputPortWidth=3  IndexOptions=Index vector (dialog)  Indices=1  OutputSizes=1
  Selector2 : Selector  InputPortWidth=3  IndexOptions=Index vector (dialog)  Indices=3  OutputSizes=1
  Selector3 : Selector  InputPortWidth=3  IndexOptions=Index vector (dialog)  Indices=[1:2]  OutputSizes=1
  states : Outport
  wires:
  Data Type Conversion1/1 -> Matrix Multiply2/2
  Selector/1 -> Mux/3  "xy"
  Quaternion Validity Check/1(Valid quat) -> Quaternions to Direction Cosine Matrix/1, Quaternions to Rotation Angles/1
  Data Type Conversion/1 -> Quaternion Validity Check/1(In1)
  Quaternions to Direction Cosine Matrix/1 -> Matrix Multiply2/1
  Selector1/1 -> Mux/4  "psi"
  Quaternions to Rotation Angles/1 -> Selector1/1  "PsiThetaPhi"
  xyyaw/1 -> Selector/1
  Quaternion/1 -> Data Type Conversion/1
  Matrix Multiply2/1 -> Selector3/1  "uvw"
  pqr/1 -> Selector2/1
  Current Velocity/1 -> Data Type Conversion1/1
  Mux/1 -> states/1  "states"
  Selector2/1 -> Mux/2  "r"
  Selector3/1 -> Mux/1  "uv"

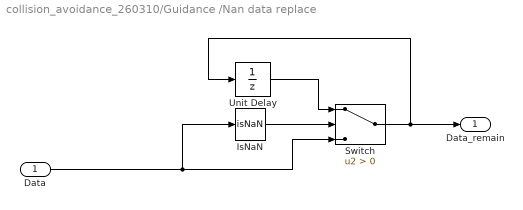
== system collision_avoidance_260310/Guidance /Nan data replace ==
  Data : Inport
  IsNaN : RelationalOperator  Operator=isNaN  OutDataTypeStr=boolean  RndMeth=Simplest  InputSameDT=off
  Switch : Switch  Criteria=u2 > Threshold  SaturateOnIntegerOverflow=off  InputSameDT=off
  Unit Delay : UnitDelay  InitialCondition=1  SampleTime=-1  HasFrameUpgradeWarning=on
  Data_remain : Outport
  wires:
  Switch/1 -> Data_remain/1, Unit Delay/1
  Data/1 -> IsNaN/1, Switch/3
  IsNaN/1 -> Switch/2
  Unit Delay/1 -> Switch/1

== system collision_avoidance_260310/Estimator Output/Input Allocation/Quaternion Validity Check ==
  In1 : Inport
  Constant : Constant  Value=[1 0 0 0]  SampleTime=-1
  Quaternion Norm : sharedutil/Quaternion Norm  aMode=aMode
  Switch : Switch  Criteria=u2 > Threshold  SaturateOnIntegerOverflow=off  InputSameDT=off
  Valid quat : Outport
  wires:
  In1/1 -> Quaternion Norm/1, Switch/1
  Quaternion Norm/1 -> Switch/2
  Switch/1 -> Valid quat/1
  Constant/1 -> Switch/3

== matlab function collision_avoidance_260310/Estimator Output/MATLAB Function ==
  data: n_loc output; e_loc output; Lat input; Lon input; ref_lla input
function [n_loc, e_loc] = global2local(Lat, Lon, ref_lla)
    % 입력:
    % Lat, Lon     : 변환할 점의 위도, 경도
    % ref_lla : 기준점 (NED 기준점, alt는 일반적으로 0으로 둠)
    
    lla = [Lat, Lon, 0];              % 변환할 점
    
    ned = lla2ned(lla, ref_lla, 'ellipsoid');  % 또는 'flat' 사용 가능
    n_loc = ned(1);  % North
    e_loc = ned(2);  % East
end

== matlab function collision_avoidance_260310/Guidance /Atan2_guidance ==
  data: u_ref output; pn input; psi_ref output; x_ref output; y_ref output; pe input; wp_north input; wp_east input; u_setpoint input; curr_index input; Total_wp input; mission_done input
function [u_ref, psi_ref, x_ref, y_ref] = Atan2_guidance( ...
    pn, pe, wp_north, wp_east, u_setpoint, curr_index, Total_wp, mission_done)

% Atan2_guidance
% curr_index : current target waypoint index from WaypointSequencer

    % default outputs
    u_ref     = u_setpoint;

    % protect empty case
    if Total_wp <= 0
        x_ref = pn;
        y_ref = pe;
        psi_ref = 0;
        u_ref = 0;
        return;
    end

    % bound index
    idx = max(1, curr_index);
    idx = min(idx, Total_wp);

    % target waypoint
    x_ref = wp_north(idx);
    y_ref = wp_east(idx);

    % heading reference
    n_diff = x_ref - pn;
    e_diff = y_ref - pe;
    psi_ref = atan2(e_diff, n_diff);

    % mission complete
    if mission_done == 1
        u_ref = 0;
    end

end

== matlab function collision_avoidance_260310/Controller/Heading Controller/MATLAB Function ==
  data: psi input; psi_mod output
function psi_mod = wrapToPi(psi)

psi_mod = mod(psi + pi, 2*pi) - pi;

== matlab function collision_avoidance_260310/Estimator Output/MATLAB Function1 ==
  data: prev_ne output; cur_ne output; Lat input; Lon input; ref_lla input
function [prev_ne, cur_ne] = globals2locals(Lat, Lon, ref_lla)
    % 입력:
    % Lat, Lon     : [lat1; lat2], [lon1; lon2] (2x1 벡터)
    % ref_lla : 기준점 (LLA 좌표계 기준) [ref_lat, ref_lon, ref_alt]
    
    % 고도 0으로 설정된 LLA 좌표
    lla1 = [Lat(1), Lon(1), 0];
    lla2 = [Lat(2), Lon(2), 0];
    
    % 각각 NED 변환
    ned1 = lla2ned(lla1, ref_lla, 'ellipsoid');
    ned2 = lla2ned(lla2, ref_lla, 'ellipsoid');
    
    % North-East만 반환
    prev_ne = [ned1(1), ned1(2)];
    cur_ne  = [ned2(1), ned2(2)];
end
